simulink model "step3"  (R2021b)
settings: Solver=VariableStepAuto  StartTime=0.0  StopTime=10.0  RelTol=1e-3
settings Model: Creator=just cookie file  LastModifiedBy=just cookie file

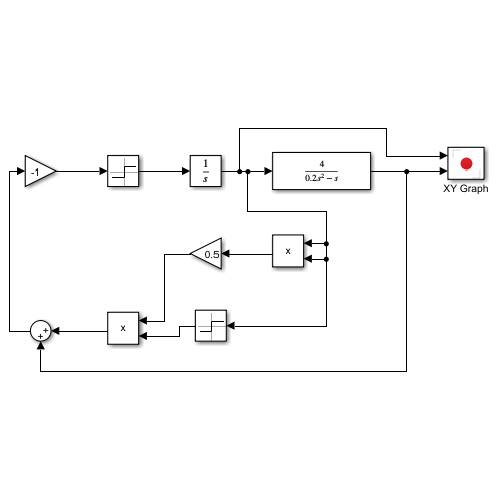
[thumbnail: Simulink's stored preview of the top-level diagram]
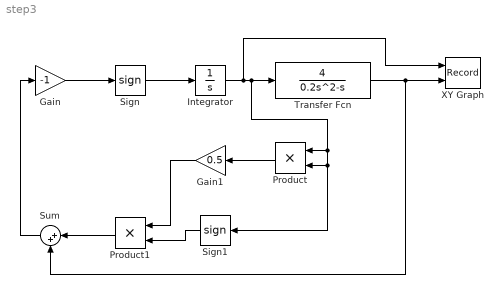
== system step3 ==
  Gain : Gain  Gain=-1
  Gain1 : Gain  Gain=0.5
  Integrator : Integrator  InitialCondition=1
  Product : Product
  Product1 : Product
  Sign : Signum
  Sign1 : Signum
  Sum : Sum  Inputs=|++
  Transfer Fcn : TransferFcn  Numerator=[4]  Denominator=[0.2 -1 0]
  XY Graph : Record  FileSettingsInternal="{\"entries\":[{\"content\":{\"excelSettings\":{\"content\":{},\"type\":\"Streamout.ExcelSettings\"}},\"type\":\"Streamout.FileSettingStorage\",\"uuid\":\"c8f97f76-8aca-4c8a-98d0-985f608419e3\"}],\"packageUris\":[\"http://schema.mathworks.com/mf0/streamout_blocks/R2020a\"],\"version\":\"1.0\"}"  Layout=[1 1]  SignalsInternal="{\"entries\":[{\"content\":{\"signals\":[{\"content\":{\"blockPath\":[\"untitled/XY Graph\"],\"channel\":[],\"dimensions\":[1],\"domain\":\"untitled/XY Graph\",\"lineColor\":\"#a2142f\",\"plots\":[1],\"port\":1,\"sid\":[\"\"],\"signalID\":245,\"signalName\":\"Integrator\"},\"type\":\"RecordBlkView.Signal\",\"uuid\":\"818ff269-9c19-4fa2-aa9a-a187e7053211\"},{\"content\":{\"blockPath\":[\"untitled/XY Graph\"],\"channel\":[],\"dimensions\":[1],\"domain\":\"untitled/XY Graph\",\"lineColor\":\"#139fff\",\"plots\":[1],\"port\":2,\"sid\":[\"\"],\"signalID\":249,\"signalName\":\"Transfer Fcn\"},\"type\":\"RecordBlkView.Signal\",\"uuid\":\"dee91938-730c-4d9b-ad2b-6bfeed1d0344\"}]},\"type\":\"RecordBlkView.InputSignals\",\"uuid\":\"7ff37d25-ccb4-491e-a72d-a328cb4946d2\"}],\"packageUris\":[\"http://schema.mathworks.com/mf0/streamout_blocks/R2020a\"],\"version\":\"1.0\"}"  VisualizationBindings="{\"xyplotplugin\":{\"info\":[{\"series\":[{\"bindingParametersList\":[{\"parameter\":\"X-Axis\",\"signalID\":245,\"signalName\":\"Integrator\"},{\"parameter\":\"Y-Axis\",\"signalID\":249,\"signalName\":\"Transfer Fcn\"}],\"seriesID\":39876}],\"subplotID\":1}]}}"  CompatibilityTag=XY
  wires:
  Sum/1 -> Gain/1
  Gain/1 -> Sign/1
  Sign/1 -> Integrator/1
  Integrator/1 -> Transfer Fcn/1, Product/2, Sign1/1, Product/1, XY Graph/1
  Transfer Fcn/1 -> Sum/2, XY Graph/2
  Product/1 -> Gain1/1
  Product1/1 -> Sum/1
  Sign1/1 -> Product1/2
  Gain1/1 -> Product1/1
